simulink model "project_Assignment"  (R2017a)
settings: Solver=FixedStepAuto  StartTime=0.0  StopTime=2  FixedStep=0.01  RelTol=1e-3
values from neighbouring files (symbols this model uses):
  A = [0 1 0 0 ... (first row only)    [Final_Project.m]
  B = [0; (-h2+(h4*h5))/((h1*h5)-h2^2); 0; ((h2^2-h4*h5*h2)/(h1*h5^2-h2^2*h5))+1/h5]    [Final_Project.m]
  C = [1 0 0 0; 0 0 1 0]    [Final_Project.m]
  D = [0;0]    [Final_Project.m]
  KvalueCT = place(A,B,pole)    [Final_Project.m]
  LvalueCT = place(A',C',Lpole)'    [Final_Project.m]
settings Model: Creator=daksh  LastModifiedBy=daksh

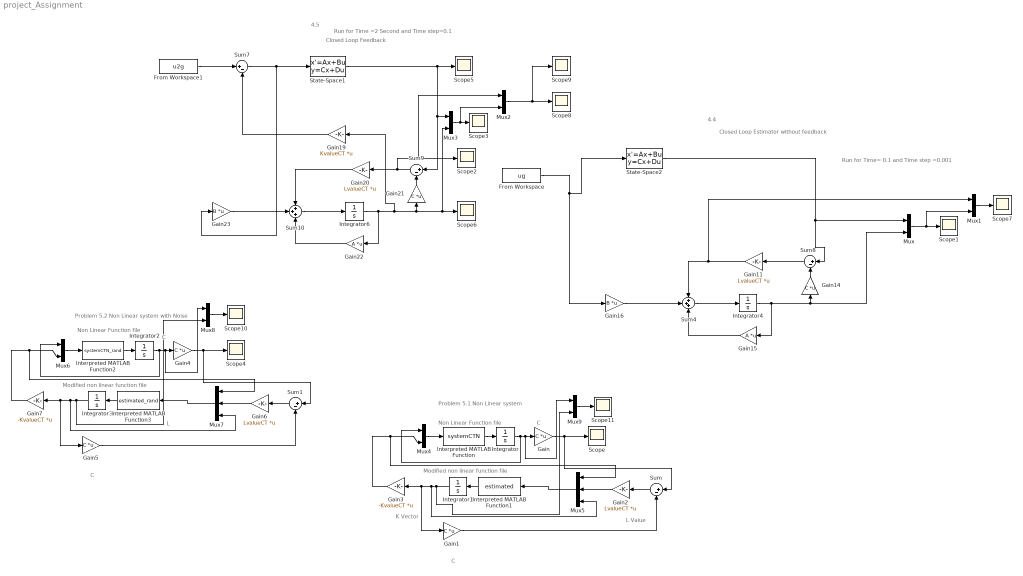
== system project_Assignment ==
  note: L Value
  note: K Vector
  note: Problem 5.2 Non Linear system with Noise
  note: Problem 5.1 Non Linear system
  note: Run for Time= 0.1 and Time step =0.001
  note: Run for Time =2 Second and Time step=0.1
  note: Closed Loop Feedback
  note: Closed Loop Estimator without feedback
  note: 4.5
  note: 4.4
  note: Non Linear Function file
  note: Modified non linear function file
  note: C
  note: C
  note: C
  note: L
  note: C
  note: Modified non linear function file
  note: Non Linear Function file
  From Workspace : FromWorkspace  VariableName=ug  SampleTime=0
  From Workspace1 : FromWorkspace  VariableName=u2g  SampleTime=0
  Gain{,1,4..5} (4 alike) : Gain  Gain=C  Multiplication=Matrix(K*u) (u vector)
  Gain11 : Gain  Gain=LvalueCT  Multiplication=Matrix(K*u)
  Gain14 : Gain  Gain=C  Multiplication=Matrix(K*u)
  Gain15 : Gain  Gain=A  Multiplication=Matrix(K*u) (u vector)
  Gain16 : Gain  Gain=B  Multiplication=Matrix(K*u)
  Gain19 : Gain  Gain=KvalueCT  Multiplication=Matrix(K*u) (u vector)
  Gain2 : Gain  Gain=LvalueCT  Multiplication=Matrix(K*u) (u vector)
  Gain20 : Gain  Gain=LvalueCT  Multiplication=Matrix(K*u)
  Gain21 : Gain  Gain=C  Multiplication=Matrix(K*u)
  Gain22 : Gain  Gain=A  Multiplication=Matrix(K*u) (u vector)
  Gain23 : Gain  Gain=B  Multiplication=Matrix(K*u)
  Gain3 : Gain  Gain=-KvalueCT  Multiplication=Matrix(K*u) (u vector)
  Gain6 : Gain  Gain=LvalueCT  Multiplication=Matrix(K*u) (u vector)
  Gain7 : Gain  Gain=-KvalueCT  Multiplication=Matrix(K*u) (u vector)
  Integrator : Integrator  InitialCondition=[pi;0;0.1;0]
  Integrator1 : Integrator  InitialCondition=[pi,0,0.1,0]
  Integrator2 : Integrator  InitialCondition=[pi;0;0.1;0]
  Integrator3 : Integrator  InitialCondition=[pi,0,0.1,0]
  Integrator4 : Integrator
  Integrator6 : Integrator
  Interpreted MATLAB Function : MATLABFcn  MATLABFcn=systemCTN
  Interpreted MATLAB Function1 : MATLABFcn  MATLABFcn=estimated
  Interpreted MATLAB Function2 : MATLABFcn  MATLABFcn=systemCTN_rand
  Interpreted MATLAB Function3 : MATLABFcn  MATLABFcn=estimated_rand
  Mux{,1..4,6,8..9} (8 alike) : Mux  Inputs=2
  Mux5 : Mux  Inputs=3
  Mux7 : Mux  Inputs=3
  Scope{,1..11} (12 alike) : Scope
  State-Space1 : StateSpace  A=A  B=B  C=C  D=D  X0=[0;0;0.1;0]
  State-Space2 : StateSpace  A=A  B=B  C=C  D=D  X0=[0.1;0.1;0.1;0.1]
  Sum{,1,7..9} (5 alike) : Sum  Inputs=|+-
  Sum10 : Sum  Inputs=+++
  Sum4 : Sum  Inputs=+++
  wires:
  Gain19/1 -> Sum7/2
  Sum7/1 -> Gain23/1, State-Space1/1
  Sum9/1 -> Mux2/1, Scope2/1, Gain20/1
  Gain22/1 -> Sum10/3
  Gain21/1 -> Sum9/2
  Integrator6/1 -> Gain22/1, Gain19/1, Mux3/2, Scope6/1, Gain21/1
  Gain20/1 -> Sum10/1
  Sum10/1 -> Integrator6/1
  Gain23/1 -> Sum10/2
  State-Space1/1 -> Scope5/1, Mux3/1, Sum9/1
  From Workspace1/1 -> Sum7/1
  Gain14/1 -> Sum8/2
  Integrator4/1 -> Gain15/1, Mux/2, Gain14/1
  Gain15/1 -> Sum4/3
  Sum8/1 -> Gain11/1
  Sum4/1 -> Integrator4/1
  Gain11/1 -> Mux1/1, Sum4/1
  State-Space2/1 -> Mux/1, Sum8/1
  Gain16/1 -> Sum4/2
  Mux/1 -> Mux1/2, Scope1/1
  From Workspace/1 -> Gain16/1, State-Space2/1
  Mux1/1 -> Scope7/1
  Mux2/1 -> Scope9/1, Scope8/1
  Mux3/1 -> Mux2/2, Scope3/1
  Integrator/1 -> Mux4/1, Mux9/1, Gain/1
  Integrator1/1 -> Mux9/2, Mux5/3, Gain1/1, Gain3/1
  Mux4/1 -> Interpreted MATLAB Function/1
  Mux5/1 -> Interpreted MATLAB Function1/1
  Gain2/1 -> Mux5/2
  Gain1/1 -> Sum/2
  Gain3/1 -> Mux4/2, Mux5/1
  Sum/1 -> Gain2/1
  Interpreted MATLAB Function1/1 -> Integrator1/1
  Gain/1 -> Sum/1, Scope/1
  Interpreted MATLAB Function/1 -> Integrator/1
  Mux6/1 -> Interpreted MATLAB Function2/1
  Sum1/1 -> Gain6/1
  Integrator2/1 -> Mux6/1, Mux8/1, Gain4/1
  Mux7/1 -> Interpreted MATLAB Function3/1
  Interpreted MATLAB Function3/1 -> Integrator3/1
  Gain4/1 -> Sum1/1, Scope4/1
  Integrator3/1 -> Mux8/2, Mux7/3, Gain5/1, Gain7/1
  Interpreted MATLAB Function2/1 -> Integrator2/1
  Gain5/1 -> Sum1/2
  Gain6/1 -> Mux7/2
  Gain7/1 -> Mux6/2, Mux7/1
  Mux8/1 -> Scope10/1
  Mux9/1 -> Scope11/1
